simulink model "sync_condenser_sim"  (R2020b)
settings: Solver=VariableStepAuto  StartTime=0.0  StopTime=10.0  RelTol=1e-3
libraries: powerlib x8, fl_lib x1
settings Model: Creator=aayushyaagarwal  LastModifiedBy=tmcnama2

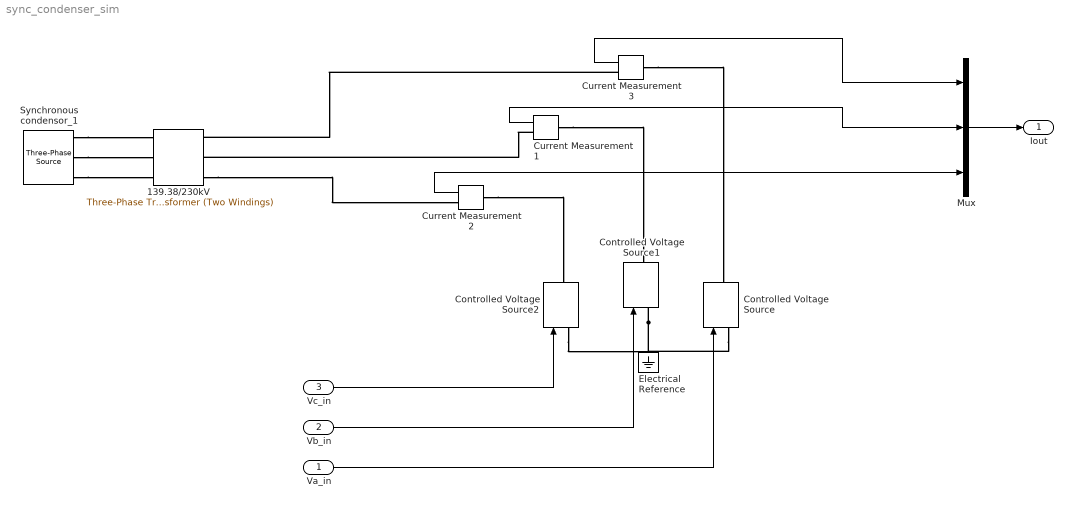
== system sync_condenser_sim ==
  Va_in : Inport
  Vb_in : Inport  Port=2
  Vc_in : Inport  Port=3
  139.38/230kV : powerlib/Elements/Three-Phase Transformer (Two Windings)  Winding1Connection=Yg  Winding2Connection=Yg  CoreType=Three single-phase transformers  SetSaturation=off  Hysteresis=off  DataFile='hysteresis'  SetInitialFlux=off  Measurements=None  UNITS=pu  NominalPower=[ 120e6 , 60 ]  Winding1=[139.38e3 , 0.002 , 0.08 ]  Winding2=[ 230e3 , 0.002 , 0.08 ]  Rm=500  Lm=500  L0=0.5  Saturation=[ 0,0 ; 0.0024,1.2 ; 1.0,1.52 ]  InitialFluxes=[ 0.8 , -0.8 , 0.7 ]  BreakLoop=off  DiscreteSolver=Trapezoidal iterative  DataType=off  TransfoNumber=1
  Controlled Voltage Source : powerlib/Electrical Sources/Controlled Voltage Source  Initialize=off  Source_Type=AC  Amplitude=0  Phase=0  Frequency=0  Measurements=Voltage
  Controlled Voltage Source1 : powerlib/Electrical Sources/Controlled Voltage Source  Initialize=off  Source_Type=AC  Amplitude=0  Phase=0  Frequency=0  Measurements=Voltage
  Controlled Voltage Source2 : powerlib/Electrical Sources/Controlled Voltage Source  Initialize=off  Source_Type=AC  Amplitude=120  Phase=0  Frequency=60  Measurements=Voltage
  Current Measurement1 : powerlib/Measurements/Current Measurement  PhasorSimulation=off  OutputType=Complex  PSBequivalent=0
  Current Measurement2 : powerlib/Measurements/Current Measurement  PhasorSimulation=off  OutputType=Complex  PSBequivalent=0
  Current Measurement3 : powerlib/Measurements/Current Measurement  PhasorSimulation=off  OutputType=Complex  PSBequivalent=0
  Electrical Reference : fl_lib/Electrical/Electrical Elements/Electrical Reference
  Mux : Mux  Inputs=3
  Synchronous condensor_1 : powerlib/Electrical Sources/Three-Phase Source  InternalConnection=Yg  VoltagePhases=off  Voltage=(139380)*1.01137  PhaseAngle=-34.48  Voltage_phases=[25e3 25e3 25e3]/sqrt(3)  PhaseAngles_phases=[0 -120 +120]  Frequency=60  NonIdealSource=on  SpecifyImpedance=off  Resistance=0.8929  Inductance=16.58e-3  ShortCircuitLevel=100e6  BaseVoltage=139.38e3  XRratio=7  BusType=PQ  Pref=0  Qref=50.096e6  Prefabc=[10e3, 10e3, 10e3]  Qrefabc=[0, 0, 0]  Qmin=-inf  Qmax=inf
  Iout : Outport  SignalName=Iout
  wires:
  Mux/1 -> Iout/1
  Vc_in/1 -> Controlled Voltage Source2/1
  Vb_in/1 -> Controlled Voltage Source1/1
  Va_in/1 -> Controlled Voltage Source/1
  Current Measurement2/1 -> Mux/3
  Current Measurement1/1 -> Mux/2
  Current Measurement3/1 -> Mux/1
  connections:
  Synchronous condensor_1/RConn3 -- 139.38/230kV/LConn3
  Synchronous condensor_1/RConn2 -- 139.38/230kV/LConn2
  Controlled Voltage Source1/LConn1 -- Controlled Voltage Source2/LConn1 -- Controlled Voltage Source/LConn1
  Synchronous condensor_1/RConn1 -- 139.38/230kV/LConn1
  Current Measurement2/LConn1 -- Controlled Voltage Source2/RConn1
  139.38/230kV/RConn3 -- Current Measurement2/RConn1
  Current Measurement1/RConn1 -- 139.38/230kV/RConn2
  Current Measurement1/LConn1 -- Controlled Voltage Source1/RConn1
  Current Measurement3/LConn1 -- Controlled Voltage Source/RConn1
  Current Measurement3/RConn1 -- 139.38/230kV/RConn1
